simulink model "phase_2"  (R2020b)
settings: Solver=VariableStepAuto  StartTime=0.0  StopTime=10.0  RelTol=1e-3
values from neighbouring files (symbols this model uses):
  A = [0 -pi/16 0;pi/16 0 3*pi/16;0 0 0]    [feedbackControllerFinal.m]
  B = [1/2 1/2;0 0;1/0.15 -1/0.15]    [feedbackControllerFinal.m]
  C = [1 0 0;0 1 0]    [feedbackControllerFinal.m]
  G_closeLoop = inv(C*inv(-(A-B*K1))*B)    [feedbackControllerFinal.m]
  K1 = place(A, B, [-30 -1+4.899*i -1-4.899*i])    [feedbackControllerFinal.m]
  K_f = K_bar(:,1:3)    [feedbackControllerFinal.m]
  Ka = K_bar(:,4:5)    [feedbackControllerFinal.m]
settings Model: Creator=BALUCH  LastModifiedBy=BALUCH

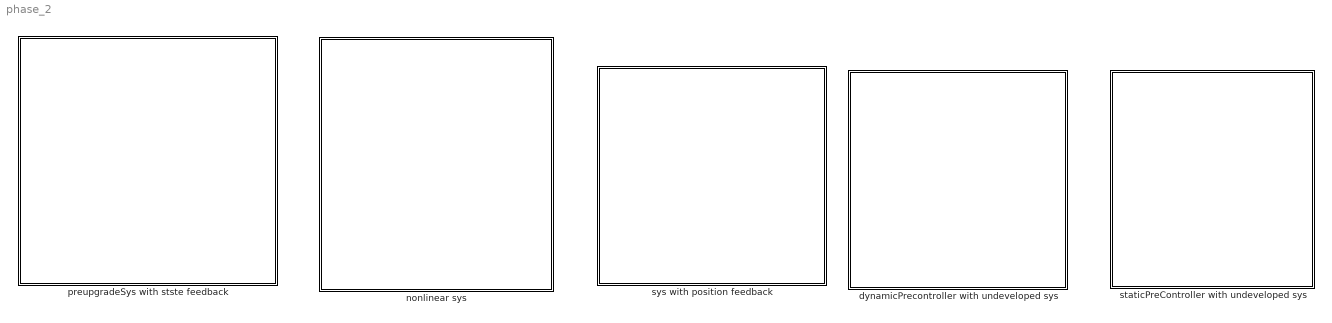
== system phase_2 ==
  "dynamicPrecontroller with undeveloped sys " : Subsystem
  "nonlinear sys " : Subsystem
  "preupgradeSys with stste feedback " : Subsystem
  staticPreController with undeveloped sys : Subsystem
  sys with position feedback : Subsystem

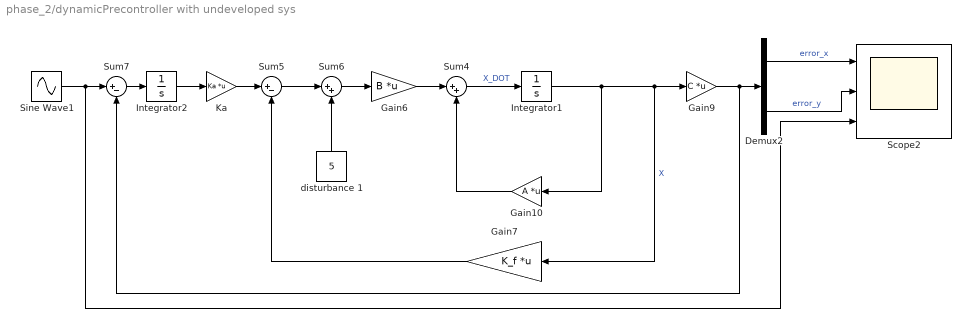
== system phase_2/dynamicPrecontroller with undeveloped sys  ==
  Demux2 : Demux  Outputs=2
  Gain10 : Gain  Gain=A  Multiplication=Matrix(K*u)
  Gain6 : Gain  Gain=B  Multiplication=Matrix(K*u)
  Gain7 : Gain  Gain=K_f  Multiplication=Matrix(K*u)
  Gain9 : Gain  Gain=C  Multiplication=Matrix(K*u)
  Integrator1 : Integrator
  Integrator2 : Integrator
  "Ka " : Gain  Gain=Ka  Multiplication=Matrix(K*u)
  Scope2 : Scope  NumInputPorts=3
  Sine Wave1 : Sin  Amplitude=[1 1]  Bias=[0 0]  Frequency=[1 1]  SampleTime=0
  Sum4 : Sum  Inputs=|++
  Sum5 : Sum  Inputs=|+-
  Sum6 : Sum  Inputs=|++
  Sum7 : Sum  Inputs=|+-
  disturbance 1 : Constant  Value=5
  wires:
  Sum5/1 -> Sum6/1
  Integrator2/1 -> "Ka "/1
  Sum7/1 -> Integrator2/1
  disturbance 1/1 -> Sum6/2
  Integrator1/1 -> Gain10/1, Gain7/1, Gain9/1  "X"
  Gain7/1 -> Sum5/2
  Gain6/1 -> Sum4/1
  Gain10/1 -> Sum4/2
  Sine Wave1/1 -> Scope2/3, Sum7/1
  Demux2/2 -> Scope2/2  "error_y"
  "Ka "/1 -> Sum5/1
  Sum6/1 -> Gain6/1
  Demux2/1 -> Scope2/1  "error_x"
  Gain9/1 -> Sum7/2, Demux2/1
  Sum4/1 -> Integrator1/1  "X_DOT"

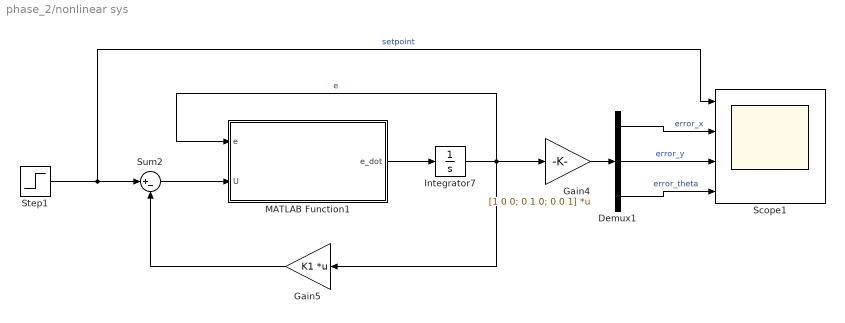
== system phase_2/nonlinear sys  ==
  Demux1 : Demux  Outputs=3
  Gain4 : Gain  Gain=[1 0 0; 0 1 0; 0 0 1]  Multiplication=Matrix(K*u)
  Gain5 : Gain  Gain=K1  Multiplication=Matrix(K*u)
  Integrator7 : Integrator  InitialCondition=[0.45; -0.3; -0.3]
  MATLAB Function1 : MATLAB Function  TreatAsAtomicUnit=on
  Scope1 : Scope  NumInputPorts=4
  Step1 : Step  Time=[0;0]  Before=[0;0]  After=[0.1;0.2]  SampleTime=0
  Sum2 : Sum  Inputs=|+-
  wires:
  Sum2/1 -> MATLAB Function1/2(U)
  Gain5/1 -> Sum2/2
  Integrator7/1 -> MATLAB Function1/1(e), Gain4/1, Gain5/1  "e"
  MATLAB Function1/1(e_dot) -> Integrator7/1
  Gain4/1 -> Demux1/1
  Demux1/1 -> Scope1/2  "error_x"
  Step1/1 -> Sum2/1, Scope1/1  "setpoint"
  Demux1/2 -> Scope1/3  "error_y"
  Demux1/3 -> Scope1/4  "error_theta"

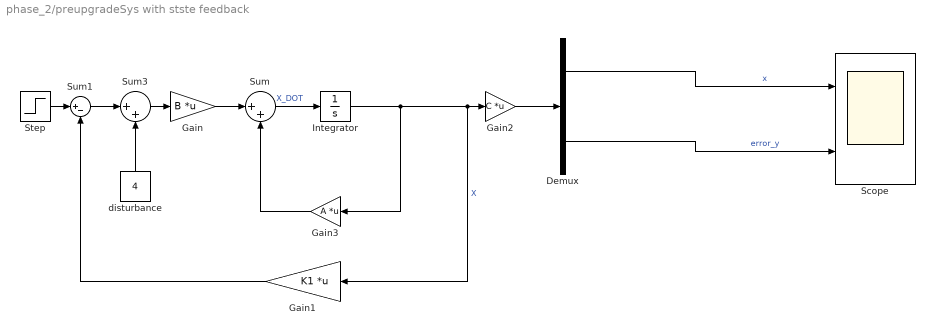
== system phase_2/preupgradeSys with stste feedback  ==
  Demux : Demux  Outputs=2
  Gain : Gain  Gain=B  Multiplication=Matrix(K*u)
  Gain1 : Gain  Gain=K1  Multiplication=Matrix(K*u)
  Gain2 : Gain  Gain=C  Multiplication=Matrix(K*u)
  Gain3 : Gain  Gain=A  Multiplication=Matrix(K*u)
  Integrator : Integrator
  Scope : Scope  NumInputPorts=2
  Step : Step  SampleTime=0
  Sum : Sum  Inputs=|++
  Sum1 : Sum  Inputs=|+-
  Sum3 : Sum  Inputs=|++
  "disturbance " : Constant  Value=4
  wires:
  Gain3/1 -> Sum/2
  Sum/1 -> Integrator/1  "X_DOT"
  Sum3/1 -> Gain/1
  Gain/1 -> Sum/1
  Gain1/1 -> Sum1/2
  "disturbance "/1 -> Sum3/2
  Integrator/1 -> Gain3/1, Gain1/1, Gain2/1  "X"
  Gain2/1 -> Demux/1
  Sum1/1 -> Sum3/1
  Step/1 -> Sum1/1
  Demux/1 -> Scope/1  "x"
  Demux/2 -> Scope/2  "error_y"

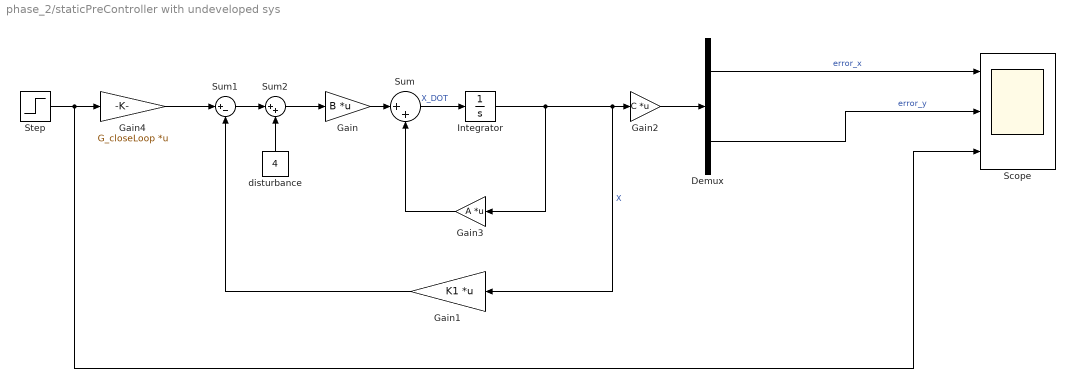
== system phase_2/staticPreController with undeveloped sys ==
  Demux : Demux  Outputs=2
  Gain : Gain  Gain=B  Multiplication=Matrix(K*u)
  Gain1 : Gain  Gain=K1  Multiplication=Matrix(K*u)
  Gain2 : Gain  Gain=C  Multiplication=Matrix(K*u)
  Gain3 : Gain  Gain=A  Multiplication=Matrix(K*u)
  Gain4 : Gain  Gain=G_closeLoop  Multiplication=Matrix(K*u)
  Integrator : Integrator
  Scope : Scope  NumInputPorts=3
  Step : Step  Time=[0 0]'  Before=[0 0]'  After=[0.8 0.4]'  SampleTime=0
  Sum : Sum  Inputs=|++
  Sum1 : Sum  Inputs=|+-
  Sum2 : Sum  Inputs=|++
  "disturbance " : Constant  Value=4
  wires:
  Gain2/1 -> Demux/1
  Gain1/1 -> Sum1/2
  Integrator/1 -> Gain2/1, Gain1/1, Gain3/1  "X"
  Gain/1 -> Sum/1
  Sum/1 -> Integrator/1  "X_DOT"
  Gain3/1 -> Sum/2
  "disturbance "/1 -> Sum2/2
  Sum1/1 -> Sum2/1
  Sum2/1 -> Gain/1
  Demux/1 -> Scope/1  "error_x"
  Demux/2 -> Scope/2  "error_y"
  Gain4/1 -> Sum1/1
  Step/1 -> Scope/3, Gain4/1

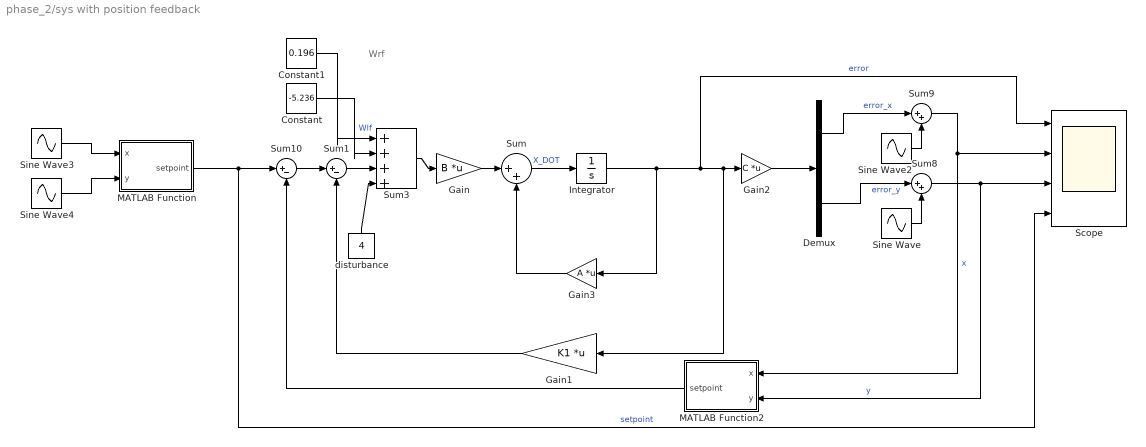
== system phase_2/sys with position feedback ==
  note: Wrf
  Constant : Constant  Value=-5.236
  Constant1 : Constant  Value=0.196
  Demux : Demux  Outputs=2
  Gain : Gain  Gain=B  Multiplication=Matrix(K*u)
  Gain1 : Gain  Gain=K1  Multiplication=Matrix(K*u)
  Gain2 : Gain  Gain=C  Multiplication=Matrix(K*u)
  Gain3 : Gain  Gain=A  Multiplication=Matrix(K*u)
  Integrator : Integrator  InitialCondition=[0.1; 0.1; 0.1]
  MATLAB Function : MATLAB Function  TreatAsAtomicUnit=on
  MATLAB Function2 : MATLAB Function  TreatAsAtomicUnit=on
  Scope : Scope  NumInputPorts=4
  Sine Wave : Sin  Amplitude=-3  Frequency=pi/16  SampleTime=0
  Sine Wave2 : Sin  Amplitude=3  Frequency=pi/16  Phase=pi/2  SampleTime=0
  Sine Wave3 : Sin  Amplitude=3  Frequency=pi/16  Phase=pi/2  SampleTime=0
  Sine Wave4 : Sin  Amplitude=-3  Frequency=pi/16  SampleTime=0
  Sum : Sum  Inputs=|++
  Sum1 : Sum  Inputs=|+-
  Sum10 : Sum  Inputs=|+-
  Sum3 : Sum  Inputs=|++++
  Sum8 : Sum  Inputs=|++
  Sum9 : Sum  Inputs=|++
  "disturbance " : Constant  Value=4
  wires:
  Demux/2 -> Sum8/1  "error_y"
  MATLAB Function2/1(setpoint) -> Sum10/2
  Constant1/1 -> Sum3/1
  Sine Wave2/1 -> Sum9/2
  Sine Wave3/1 -> MATLAB Function/1(x)
  Sine Wave4/1 -> MATLAB Function/2(y)
  Constant/1 -> Sum3/2  "Wlf"
  Sum1/1 -> Sum3/3
  Sum/1 -> Integrator/1  "X_DOT"
  Sine Wave/1 -> Sum8/2
  Sum3/1 -> Gain/1
  "disturbance "/1 -> Sum3/4
  Gain1/1 -> Sum1/2
  Gain/1 -> Sum/1
  Integrator/1 -> Gain2/1, Gain1/1, Scope/1, Gain3/1  "error"
  MATLAB Function/1(setpoint) -> Sum10/1, Scope/4  "setpoint"
  Sum10/1 -> Sum1/1
  Gain2/1 -> Demux/1
  Sum8/1 -> Scope/3, MATLAB Function2/2(y)  "y"
  Gain3/1 -> Sum/2
  Sum9/1 -> Scope/2, MATLAB Function2/1(x)  "x"
  Demux/1 -> Sum9/1  "error_x"

== matlab function phase_2/sys with position feedback/MATLAB Function ==
  data: x input; setpoint output; y input
function setpoint = fcn(x, y)

setpoint = [x; y];

== matlab function phase_2/sys with position feedback/MATLAB Function2 ==
  data: x input; setpoint output; y input
function setpoint = fcn(x, y)

setpoint = [x; y];

== matlab function phase_2/nonlinear sys /MATLAB Function1 ==
  data: e input; U input; e_dot output
function e_dot  = fcn(e,U)
e_dot = [0.1;-0.1;0.05]; 
theta_dot_ref = -(pi/16) ;
v_ref = 3*(pi/16) ;
e_dot(1)=(theta_dot_ref - U(1))*e(2) + v_ref*cos(e(3))+(U(2) - v_ref);
e_dot(2)=(U(1)-theta_dot_ref)*e(1) + v_ref*sin(e(3));
e_dot(3)= U(1);
